simulink model "assignment4"  (R2019a)
settings: Solver=FixedStepDiscrete  StartTime=0.0  StopTime=10.0  RelTol=1e-3
libraries: simulink x1
settings Model: Creator=INDIA  LastModifiedBy=INDIA

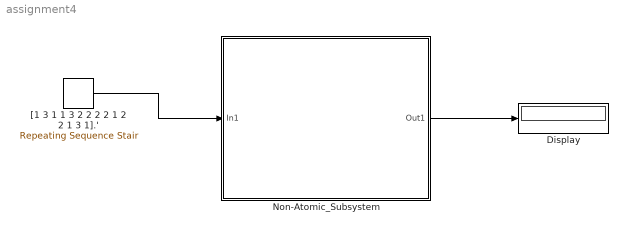
== system assignment4 ==
  Display : Display
  Non-Atomic_Subsystem : Subsystem
  "[1 3 1 1 3 2 2 2 2 1 2 2 1 3 1].'" : simulink/Sources/Repeating Sequence Stair  OutValues=[1 3 1 1 3 2 2 2 2 1 2 2 1 3 1].'  tsamp=-1  OutMin=[]  OutMax=[]  OutDataTypeStr=double  OutputDataTypeScalingMode=double  OutDataType=fixdt(0,8)  ConRadixGroup=Best Precision: Vector-wise  OutScaling=2^-12
  wires:
  "[1 3 1 1 3 2 2 2 2 1 2 2 1 3 1].'"/1 -> Non-Atomic_Subsystem/1(In1)
  Non-Atomic_Subsystem/1(Out1) -> Display/1

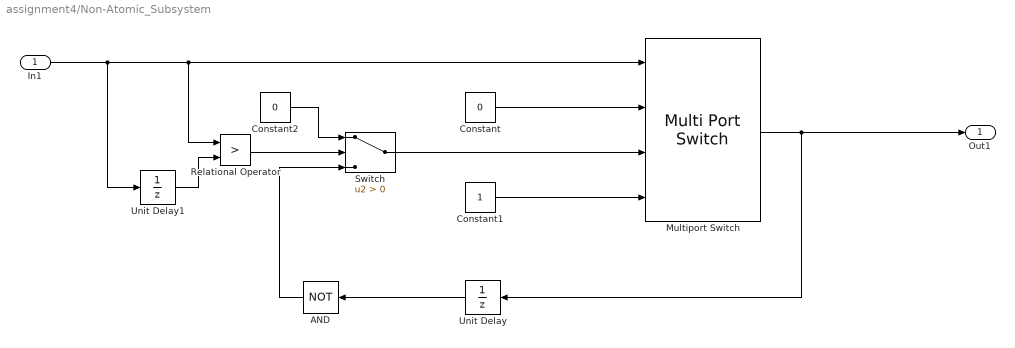
== system assignment4/Non-Atomic_Subsystem ==
  In1 : Inport
  AND : Logic  Operator=NOT  IconShape=distinctive  AllPortsSameDT=off  OutDataTypeStr=boolean
  Constant : Constant  Value=0
  Constant1 : Constant
  Constant2 : Constant  Value=0
  Multiport Switch : MultiPortSwitch
  Relational Operator : RelationalOperator  Operator=>  OutDataTypeStr=boolean  RndMeth=Simplest
  Switch : Switch  Criteria=u2 > Threshold
  Unit Delay : UnitDelay  SampleTime=-1  HasFrameUpgradeWarning=on
  Unit Delay1 : UnitDelay  SampleTime=-1  HasFrameUpgradeWarning=on
  Out1 : Outport
  wires:
  Constant/1 -> Multiport Switch/2
  In1/1 -> Unit Delay1/1, Relational Operator/1, Multiport Switch/1
  Multiport Switch/1 -> Out1/1, Unit Delay/1
  Constant2/1 -> Switch/1
  AND/1 -> Switch/3
  Unit Delay/1 -> AND/1
  Constant1/1 -> Multiport Switch/4
  Unit Delay1/1 -> Relational Operator/2
  Switch/1 -> Multiport Switch/3
  Relational Operator/1 -> Switch/2
